simulink model "quaternion_test"  (R2021a)
settings: Solver=VariableStepAuto  StartTime=0.0  StopTime=10.0  RelTol=1e-3
libraries: sharedtransform x6, sharedutil x1
settings Model: Creator=DELL  LastModifiedBy=DELL

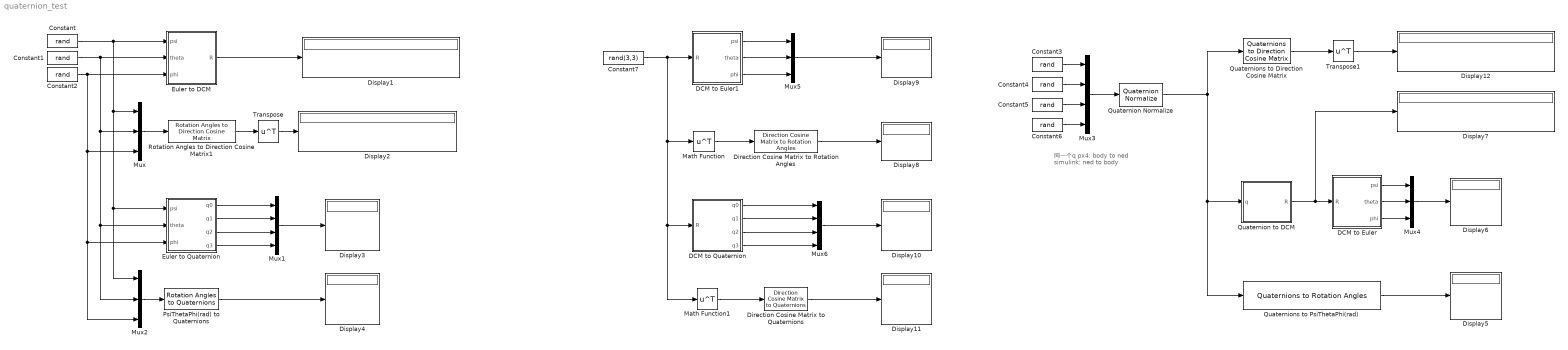
== system quaternion_test ==
  note: 同一个q
      | px4:        body to ned
      | simulink: ned to body
  Constant{,1..6} (7 alike) : Constant  Value=rand
  Constant7 : Constant  Value=rand(3,3)
  DCM to Euler : MATLAB Function  TreatAsAtomicUnit=on
  DCM to Euler1 : MATLAB Function  TreatAsAtomicUnit=on
  DCM to Quaternion : MATLAB Function  TreatAsAtomicUnit=on
  Direction Cosine Matrix to Rotation Angles : sharedtransform/Direction Cosine Matrix to Rotation Angles  rotationOrder=ZYX  aMode=aMode  action=None  tolerance=eps(2)
      settings: SourceProductBaseCode=AE,PW,DR,MT,UV,VE
  Direction Cosine Matrix to Quaternions : sharedtransform/Direction Cosine Matrix  to Quaternions  aMode=0  action=None  tolerance=eps(2)
      settings: SourceProductBaseCode=AE,PW,DR,MT,UV,VE
  Display{1..12} (12 alike) : Display
  Euler to DCM : MATLAB Function  TreatAsAtomicUnit=on
  Euler to Quaternion : MATLAB Function  TreatAsAtomicUnit=on
  Math Function : Math  Operator=transpose  SaturateOnIntegerOverflow=on
  Math Function1 : Math  Operator=transpose  SaturateOnIntegerOverflow=on
  Mux{,2,4..5} (4 alike) : Mux  Inputs=3
  Mux1 : Mux
  Mux3 : Mux
  Mux6 : Mux
  PsiThetaPhi(rad) to Quaternions : sharedtransform/Rotation Angles to Quaternions  rotationOrder=ZYX  aMode=aMode
      settings: SourceProductBaseCode=AE,PW,DR,MT,UV,VE
  Quaternion Normalize : sharedutil/Quaternion Normalize  aMode=aMode
      settings: SourceProductBaseCode=AE,PW,DR,MT,UV,VE
  Quaternion to DCM : MATLAB Function  TreatAsAtomicUnit=on
  Quaternions to Direction Cosine Matrix : sharedtransform/Quaternions to  Direction Cosine Matrix  aMode=aMode
      settings: SourceProductBaseCode=AE,PW,DR,MT,UV,VE
  Quaternions to PsiThetaPhi(rad) : sharedtransform/Quaternions to Rotation Angles  rotationOrder=ZYX  aMode=aMode
      settings: SourceProductBaseCode=AE,PW,DR,MT,UV,VE
  Rotation Angles to Direction Cosine Matrix1 : sharedtransform/Rotation Angles to Direction Cosine Matrix  rotationOrder=ZYX  aMode=aMode
      settings: SourceProductBaseCode=AE,PW,DR,MT,UV,VE
  Transpose : Math  Operator=transpose  SaturateOnIntegerOverflow=on
  Transpose1 : Math  Operator=transpose  SaturateOnIntegerOverflow=on
  wires:
  DCM to Euler/1(psi) -> Mux4/1
  DCM to Euler/3(phi) -> Mux4/3
  Quaternion to DCM/1(R) -> Display7/1, DCM to Euler/1(R)
  DCM to Euler/2(theta) -> Mux4/2
  Mux4/1 -> Display6/1
  Mux/1 -> Rotation Angles to Direction Cosine Matrix1/1
  Constant/1 -> Euler to DCM/1(psi), Mux2/1, Euler to Quaternion/1(psi), Mux/1
  Constant1/1 -> Euler to DCM/2(theta), Mux2/2, Euler to Quaternion/2(theta), Mux/2
  Constant2/1 -> Mux2/3, Euler to Quaternion/3(phi), Mux/3, Euler to DCM/3(phi)
  Rotation Angles to Direction Cosine Matrix1/1 -> Transpose/1
  Euler to DCM/1(R) -> Display1/1
  Transpose/1 -> Display2/1
  Euler to Quaternion/1(q0) -> Mux1/1
  Euler to Quaternion/2(q1) -> Mux1/2
  Euler to Quaternion/3(q2) -> Mux1/3
  Euler to Quaternion/4(q3) -> Mux1/4
  Mux1/1 -> Display3/1
  PsiThetaPhi(rad) to Quaternions/1 -> Display4/1
  Mux2/1 -> PsiThetaPhi(rad) to Quaternions/1
  Quaternions to PsiThetaPhi(rad)/1 -> Display5/1
  Constant3/1 -> Mux3/1
  Constant4/1 -> Mux3/2
  Constant5/1 -> Mux3/3
  Constant6/1 -> Mux3/4
  Constant7/1 -> Math Function1/1, DCM to Quaternion/1(R), Math Function/1, DCM to Euler1/1(R)
  Math Function/1 -> Direction Cosine Matrix to Rotation Angles/1
  DCM to Euler1/1(psi) -> Mux5/1
  DCM to Euler1/2(theta) -> Mux5/2
  DCM to Euler1/3(phi) -> Mux5/3
  Direction Cosine Matrix to Rotation Angles/1 -> Display8/1
  Mux5/1 -> Display9/1
  DCM to Quaternion/1(q0) -> Mux6/1
  DCM to Quaternion/2(q1) -> Mux6/2
  DCM to Quaternion/3(q2) -> Mux6/3
  DCM to Quaternion/4(q3) -> Mux6/4
  Mux6/1 -> Display10/1
  Math Function1/1 -> Direction Cosine Matrix to Quaternions/1
  Direction Cosine Matrix to Quaternions/1 -> Display11/1
  Quaternions to Direction Cosine Matrix/1 -> Transpose1/1
  Transpose1/1 -> Display12/1
  Mux3/1 -> Quaternion Normalize/1
  Quaternion Normalize/1 -> Quaternions to Direction Cosine Matrix/1, Quaternions to PsiThetaPhi(rad)/1, Quaternion to DCM/1(q)

== matlab function quaternion_test/Euler to DCM ==
  data: R output; psi input; theta input; phi input
function R = fcn(psi,theta,phi)

R = zeros(3,3);

cosPhi = cos(phi);
sinPhi = sin(phi);
cosThe = cos(theta);
sinThe = sin(theta);
cosPsi = cos(psi);
sinPsi = sin(psi);

R(1, 1) = cosThe * cosPsi;
R(1, 2) = -cosPhi * sinPsi + sinPhi * sinThe * cosPsi;
R(1, 3) = sinPhi * sinPsi + cosPhi * sinThe * cosPsi;

R(2, 1) = cosThe * sinPsi;
R(2, 2) = cosPhi * cosPsi + sinPhi * sinThe * sinPsi;
R(2, 3) = -sinPhi * cosPsi + cosPhi * sinThe * sinPsi;

R(3, 1) = -sinThe;
R(3, 2) = sinPhi * cosThe;
R(3, 3) = cosPhi * cosThe;

end

== matlab function quaternion_test/DCM to Quaternion ==
  data: R input; q0 output; q1 output; q2 output; q3 output
function [q0,q1,q2,q3] = fcn(R)

t1 = R(1,1) + R(2,2) + R(3,3);

if t1 > 0
    t = sqrt(1 + t1);
    q0 = 0.5 * t;
    t = 0.5 / t;
    q1 = (R(3,2) - R(2,3)) * t;
    q2 = (R(1,3) - R(3,1)) * t;
    q3 = (R(2,1) - R(1,2)) * t;
    
elseif (R(1,1) > R(2,2)) && (R(1,1) > R(3,3))
    t = sqrt(1 + R(1,1) - R(2,2) - R(3,3));
    q1 = 0.5 * t;
    t = 0.5 / t;
    q0 = (R(3,2) - R(2,3)) * t;
    q2 = (R(2,1) + R(1,2)) * t;
    q3 = (R(1,3) + R(3,1)) * t;
    
elseif R(2,2) > R(3,3)
    t = sqrt(1 - R(1,1) + R(2,2) - R(3,3));
    q2 = 0.5 * t;
    t = 0.5 / t;
    q0 = (R(1,3) - R(3,1)) * t;
    q1 = (R(2,1) + R(1,2)) * t;
    q3 = (R(3,2) + R(2,3)) * t;
    
else
    t = sqrt(1 - R(1,1) - R(2,2) + R(3,3));
    q3 = 0.5 * t;
    t = 0.5 / t;
    q0 = (R(2,1) - R(1,2)) * t;
    q1 = (R(1,3) + R(3,1)) * t;
    q2 = (R(3,2) + R(2,3)) * t;
    
end

end

== matlab function quaternion_test/Euler to Quaternion ==
  data: q0 output; psi input; theta input; phi input; q1 output; q2 output; q3 output
function [q0,q1,q2,q3] = fcn(psi,theta,phi)

cosPhi_2 = cos(phi / 2);
cosTheta_2 = cos(theta / 2);
cosPsi_2 = cos(psi / 2);
sinPhi_2 = sin(phi / 2);
sinTheta_2 = sin(theta / 2);
sinPsi_2 = sin(psi / 2);

q0 = cosPhi_2 * cosTheta_2 * cosPsi_2 + sinPhi_2 * sinTheta_2 * sinPsi_2;
q1 = sinPhi_2 * cosTheta_2 * cosPsi_2 - cosPhi_2 * sinTheta_2 * sinPsi_2;
q2 = cosPhi_2 * sinTheta_2 * cosPsi_2 + sinPhi_2 * cosTheta_2 * sinPsi_2;
q3 = cosPhi_2 * cosTheta_2 * sinPsi_2 - sinPhi_2 * sinTheta_2 * cosPsi_2;

end

== matlab function quaternion_test/DCM to Euler1 ==
  data: psi output; theta output; phi output; R input
function [psi,theta,phi] = fcn(R)

theta = asin(-R(3,1));

if (abs(theta - pi/2)) < 1e-3
    phi = 0;
    psi = atan2(R(2, 3), R(1, 3));
    
elseif (abs(theta + pi/2)) < 1e-3
    phi = 0;
    psi = atan2(-R(2, 3), -R(1, 3));
    
else
    phi = atan2(R(3, 2), R(3, 3));
    psi = atan2(R(2, 1), R(1, 1));
    
end

end

== matlab function quaternion_test/Quaternion to DCM ==
  data: R output; q input
function R = fcn(q)

R = zeros(3,3);

a = q(1);
b = q(2);
c = q(3);
d = q(4);

aa = a * a;
ab = a * b;
ac = a * c;
ad = a * d;
bb = b * b;
bc = b * c;
bd = b * d;
cc = c * c;
cd = c * d;
dd = d * d;

R(1, 1) = aa + bb - cc - dd;
R(1, 2) = 2 * (bc - ad);
R(1, 3) = 2 * (ac + bd);
R(2, 1) = 2 * (bc + ad);
R(2, 2) = aa - bb + cc - dd;
R(2, 3) = 2 * (cd - ab);
R(3, 1) = 2 * (bd - ac);
R(3, 2) = 2 * (ab + cd);
R(3, 3) = aa - bb - cc + dd;

end

== matlab function quaternion_test/DCM to Euler ==
  data: psi output; theta output; phi output; R input
function [psi,theta,phi] = fcn(R)

theta = asin(-R(3,1));

if (abs(theta - pi/2)) < 1e-3
    phi = 0;
    psi = atan2(R(2, 3), R(1, 3));
    
elseif (abs(theta + pi/2)) < 1e-3
    phi = 0;
    psi = atan2(-R(2, 3), -R(1, 3));
    
else
    phi = atan2(R(3, 2), R(3, 3));
    psi = atan2(R(2, 1), R(1, 1));
    
end

end
